simulink model "ekviv_prenos_dcv4"  (R2018a)
settings: Solver=FixedStepAuto  StartTime=0.0  StopTime=10  FixedStep=0.01  RelTol=1e-3
values from neighbouring files (symbols this model uses):
  delta = 1    [init_dcv4.m]
  m = 0.5    [init_dcv4.m]
  M = 1    [init_dcv4.m]
settings Model: Creator=Martin  LastModifiedBy=Martin

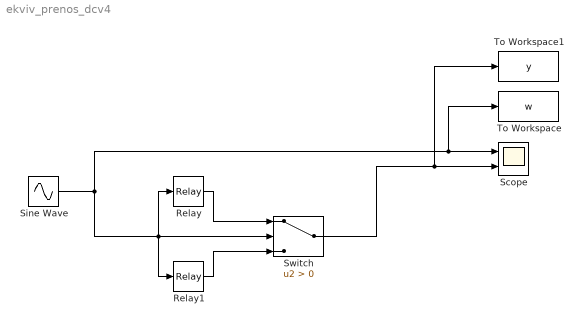
== system ekviv_prenos_dcv4 ==
  Relay : Relay  OnSwitchValue=delta  OffSwitchValue=m*delta  OnOutputValue=M
  Relay1 : Relay  OnSwitchValue=-m*delta  OffSwitchValue=-delta  OnOutputValue=0  OffOutputValue=-M
  Scope : Scope  NumInputPorts=2
  Sine Wave : Sin  Amplitude=2  Frequency=2  SampleTime=0
  Switch : Switch  Criteria=u2 > Threshold
  To Workspace : ToWorkspace  VariableName=w  SaveFormat=Timeseries  SampleTime=-1
  To Workspace1 : ToWorkspace  VariableName=y  SaveFormat=Timeseries  SampleTime=-1
  wires:
  Relay/1 -> Switch/1
  Sine Wave/1 -> Switch/2, Relay1/1, Relay/1, To Workspace/1, Scope/1
  Switch/1 -> To Workspace1/1, Scope/2
  Relay1/1 -> Switch/3
